simulink model "ComplementaryFilter"  (R2025a)
settings: Solver=VariableStepAuto  StartTime=0.0  StopTime=10.0  RelTol=1e-3
model workspace (MAT data in the model file):
  SamplingRate = 0.1
  Tuner_Main = 0.122336769759
  Tuner_Sub = 0.72
settings Model: Creator=Pablo  LastModifiedBy=Pablo

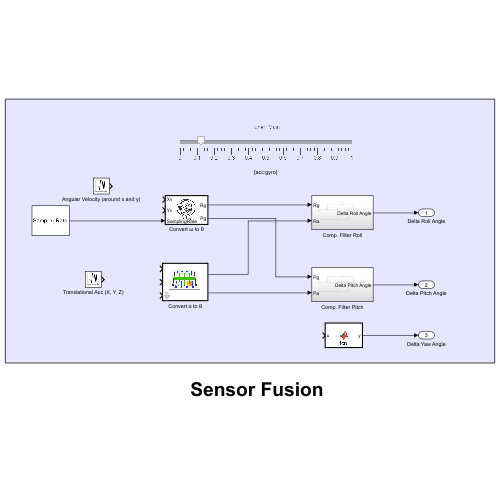
[thumbnail: Simulink's stored preview of the top-level diagram]
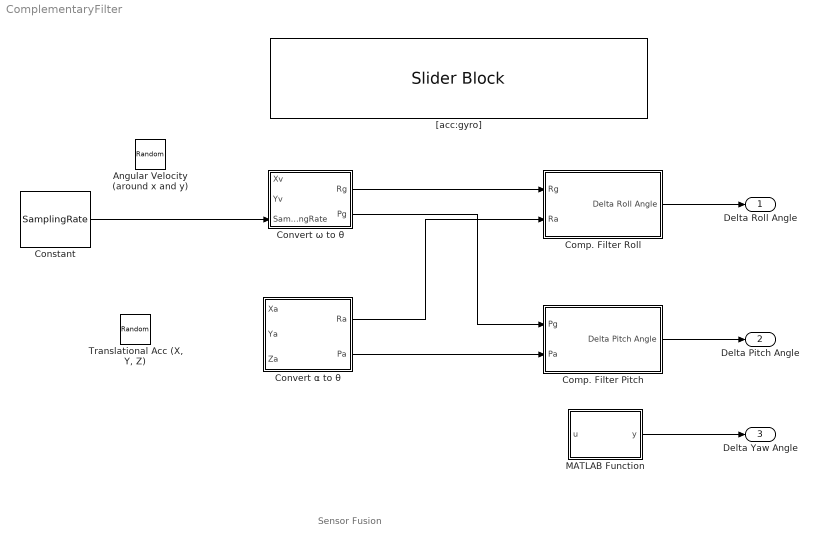
== system ComplementaryFilter ==
  note: Sensor Fusion
  Angular Velocity (around x and y) : RandomNumber  Mean=[0 0 0]  Variance=[0.1 0.1 0.1]  SampleTime=0.1
  Comp. Filter Pitch : Subsystem
  Comp. Filter Roll : Subsystem
  Constant : Constant  Value=SamplingRate
  Convert α to θ : MATLAB Function  TreatAsAtomicUnit=on
  Convert ω to θ : MATLAB Function  TreatAsAtomicUnit=on
  MATLAB Function : MATLAB Function  TreatAsAtomicUnit=on
  "Translational Acc (X, Y, Z)" : RandomNumber  Mean=[0 0 0]  Variance=[0.01 0.01 0.01]  SampleTime=0.1
  "[acc:gyro]" : SliderBlock  ScaleMax=1  TickInterval=0.1
  Delta Roll Angle : Outport
  Delta Pitch Angle : Outport  Port=2
  Delta Yaw Angle : Outport  Port=3
  wires:
  Constant/1 -> Convert ω to θ/3(SamplingRate)
  Comp. Filter Roll/1(Delta Roll Angle) -> Delta Roll Angle/1
  Comp. Filter Pitch/1(Delta Pitch Angle) -> Delta Pitch Angle/1
  Convert ω to θ/1(Rg) -> Comp. Filter Roll/1(Rg)
  Convert α to θ/1(Ra) -> Comp. Filter Roll/2(Ra)
  Convert ω to θ/2(Pg) -> Comp. Filter Pitch/1(Pg)
  Convert α to θ/2(Pa) -> Comp. Filter Pitch/2(Pa)
  MATLAB Function/1(y) -> Delta Yaw Angle/1

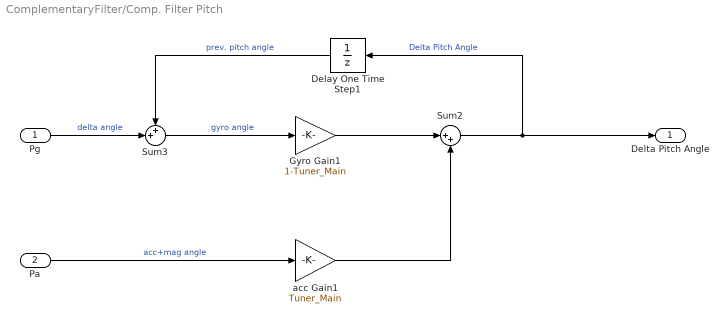
== system ComplementaryFilter/Comp. Filter Pitch ==
  Pg : Inport
  Pa : Inport  Port=2
  Delay One Time Step1 : UnitDelay  SampleTime=-1  HasFrameUpgradeWarning=on
  Gyro Gain1 : Gain  Gain=1-Tuner_Main
  Sum2 : Sum  Inputs=|++
  Sum3 : Sum  Inputs=++|
  acc Gain1 : Gain  Gain=Tuner_Main
  Delta Pitch Angle : Outport
  wires:
  Delay One Time Step1/1 -> Sum3/1  "prev. pitch angle"
  Pa/1 -> acc Gain1/1  "acc+mag angle"
  Pg/1 -> Sum3/2  "delta angle"
  Sum2/1 -> Delta Pitch Angle/1, Delay One Time Step1/1  "Delta Pitch Angle"
  acc Gain1/1 -> Sum2/2
  Gyro Gain1/1 -> Sum2/1
  Sum3/1 -> Gyro Gain1/1  "gyro angle"

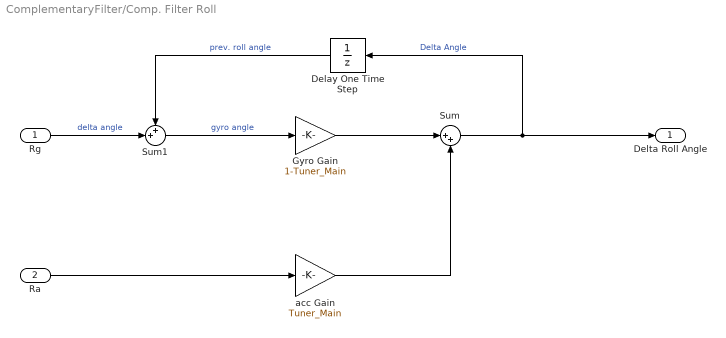
== system ComplementaryFilter/Comp. Filter Roll ==
  Rg : Inport
  Ra : Inport  Port=2
  Delay One Time Step : UnitDelay  SampleTime=-1  HasFrameUpgradeWarning=on
  Gyro Gain : Gain  Gain=1-Tuner_Main
  Sum : Sum  Inputs=|++
  Sum1 : Sum  Inputs=++|
  acc Gain : Gain  Gain=Tuner_Main
  Delta Roll Angle : Outport
  wires:
  Sum1/1 -> Gyro Gain/1  "gyro angle"
  Gyro Gain/1 -> Sum/1
  Rg/1 -> Sum1/2  "delta angle"
  Sum/1 -> Delta Roll Angle/1, Delay One Time Step/1  "Delta Angle"
  acc Gain/1 -> Sum/2
  Delay One Time Step/1 -> Sum1/1  "prev. roll angle"
  Ra/1 -> acc Gain/1

== matlab function ComplementaryFilter/Convert α to θ ==
  data: Ra output; Pa output; Xa input; Ya input; Za input
function [Ra, Pa]  = fcn(Xa, Ya, Za)

Ra = atan2d(Ya , Za);
Pa = atan2d((- Xa) , sqrt(Ya^2 + Za^2));
end

== matlab function ComplementaryFilter/Convert ω to θ ==
  data: Xv input; Rg output; Yv input; Pg output; SamplingRate input
function [Rg,Pg] = fcn(Xv, Yv, SamplingRate)
    Rg = Xv*SamplingRate;
    Pg = Yv*SamplingRate;
end

== matlab function ComplementaryFilter/MATLAB Function ==
  data: u input; y output
function y = fcn(u)

y = u;
